simulink library "MainLibrary"  (R2022b)
settings: Solver=VariableStepAuto  StartTime=0.0  StopTime=10.0  RelTol=1e-3
undefined symbols (not defined in the file or in its folder): Data, Data_SL_Info, Encoding, Encoding_SL_Info, Height, IsBigendian, Step, Width
libraries: robotlib x14, simulink_extras x2, robotcorelib x1
settings Model: Creator=20211327  LastModifiedBy=20222146

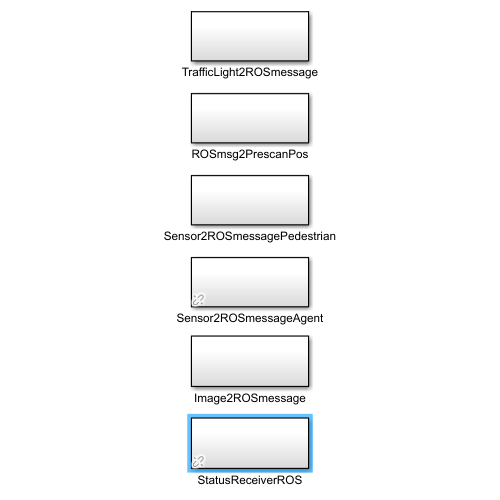
[thumbnail: Simulink's stored preview of the top-level diagram]
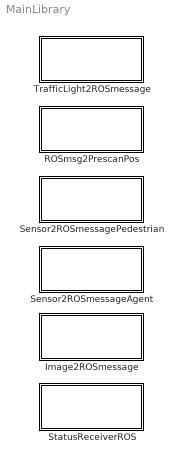
== system MainLibrary ==
  Image2ROSmessage : Subsystem
  ROSmsg2PrescanPos : Subsystem
  Sensor2ROSmessageAgent : Subsystem  AncestorBlock=MainLibrary/Sensor2ROSmessage
      settings: LibrarySourceBlock=MainLibrary/Sensor2ROSmessage
  Sensor2ROSmessagePedestrian : Subsystem
  StatusReceiverROS : Subsystem  AncestorBlock=MainLibrary/Image2ROSmessage
      settings: LibrarySourceBlock=MainLibrary/Image2ROSmessage
  TrafficLight2ROSmessage : Subsystem

== system MainLibrary/Image2ROSmessage ==
  Image Publisher : Subsystem  mask(Image publisher block){}
      mask help: This block publishes the camera image output of the experiment to a ros topic
      mask Display:
      | fprintf('Image Publisher')
      | port_label('input',1,'R')
      | port_label('input',2,'G')
      | port_label('input',3,'B')

== system MainLibrary/ROSmsg2PrescanPos ==
  ROS msg to Prescan Pos : Subsystem

== system MainLibrary/Sensor2ROSmessageAgent ==
  Sensor ROS Message Agent : Subsystem  AncestorBlock=MainLibrary/Sensor2ROSmessagePedestrian/Sensor ROS Message Pedestrian  TreatAsAtomicUnit=on
      settings: LibrarySourceBlock=MainLibrary/Sensor2ROSmessagePedestrian/Sensor ROS Message Pedestrian

== system MainLibrary/Sensor2ROSmessagePedestrian ==
  Sensor ROS Message Pedestrian : Subsystem  TreatAsAtomicUnit=on

== system MainLibrary/StatusReceiverROS ==
  Status Receiver ROS : Subsystem

== system MainLibrary/TrafficLight2ROSmessage ==
  Traffic Light ROS Message : Subsystem

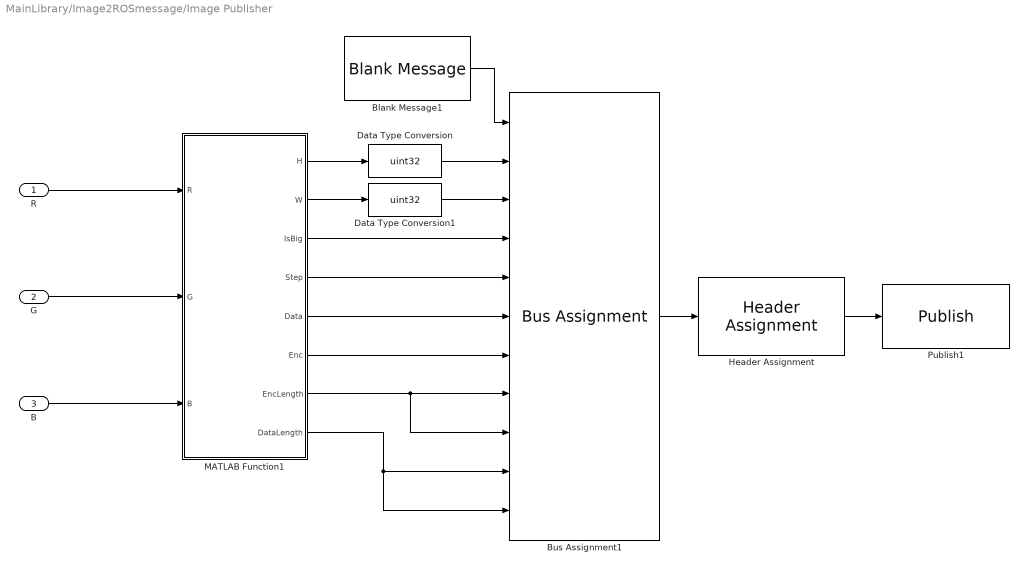
== system MainLibrary/Image2ROSmessage/Image Publisher ==
  R : Inport
  G : Inport  Port=2
  B : Inport  Port=3
  Blank Message1 : robotlib/Blank Message  messageClass=Message  entityType=sensor_msgs/Image  messageType=sensor_msgs/Image  SampleTime=inf  legacyBusStruct=off
  Bus Assignment1 : BusAssignment  AssignedSignals=Height,Width,IsBigendian,Step,Data,Encoding,Encoding_SL_Info.CurrentLength,Encoding_SL_Info.ReceivedLength,Data_SL_Info.CurrentLength,Data_SL_Info.ReceivedLength
  Data Type Conversion : DataTypeConversion  OutDataTypeStr=uint32  RndMeth=Round  SaturateOnIntegerOverflow=off
  Data Type Conversion1 : DataTypeConversion  OutDataTypeStr=uint32  RndMeth=Round  SaturateOnIntegerOverflow=off
  Header Assignment : robotlib/Header Assignment  SetFrameID=on  FrameID=camera  InsertTimeStamp=on  SetHeaderFieldName=Use the default Header field name  HeaderFieldName=Header
  MATLAB Function1 : MATLAB Function  TreatAsAtomicUnit=on
  Publish1 : robotlib/Publish  topicSource=Specify your own  topic=/camera/image  messageType=sensor_msgs/Image  legacyBusStruct=off  messageQueueLength=1
  wires:
  R/1 -> MATLAB Function1/1(R)
  G/1 -> MATLAB Function1/2(G)
  B/1 -> MATLAB Function1/3(B)
  Data Type Conversion/1 -> Bus Assignment1/2
  Data Type Conversion1/1 -> Bus Assignment1/3
  Bus Assignment1/1 -> Header Assignment/1
  Header Assignment/1 -> Publish1/1
  MATLAB Function1/4(Step) -> Bus Assignment1/5
  MATLAB Function1/7(EncLength) -> Bus Assignment1/9, Bus Assignment1/8
  MATLAB Function1/3(IsBig) -> Bus Assignment1/4
  MATLAB Function1/2(W) -> Data Type Conversion1/1
  MATLAB Function1/5(Data) -> Bus Assignment1/6
  Blank Message1/1 -> Bus Assignment1/1
  MATLAB Function1/6(Enc) -> Bus Assignment1/7
  MATLAB Function1/1(H) -> Data Type Conversion/1
  MATLAB Function1/8(DataLength) -> Bus Assignment1/11, Bus Assignment1/10

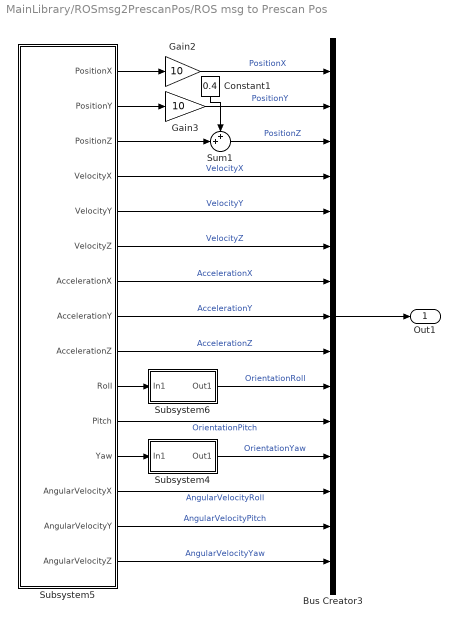
== system MainLibrary/ROSmsg2PrescanPos/ROS msg to Prescan Pos ==
  Bus Creator3 : BusCreator  Inputs=15  OutDataTypeStr=Bus: PRESCAN_STATEACTUATORDATA  NonVirtualBus=on
  Constant1 : Constant  Value=0.4
  Gain2 : Gain  Gain=10
  Gain3 : Gain  Gain=10
  Subsystem4 : Subsystem
  Subsystem5 : Subsystem
  Subsystem6 : Subsystem
  Sum1 : Sum  Inputs=++|
  Out1 : Outport
  wires:
  Subsystem5/15(AngularVelocityZ) -> Bus Creator3/15  "AngularVelocityYaw"
  Subsystem5/3(PositionZ) -> Sum1/2
  Subsystem5/7("AccelerationX ") -> Bus Creator3/7  "AccelerationX"
  Gain3/1 -> Bus Creator3/2  "PositionY"
  Subsystem5/14(AngularVelocityY) -> Bus Creator3/14  "AngularVelocityPitch"
  Subsystem5/8(AccelerationY) -> Bus Creator3/8  "AccelerationY"
  Subsystem5/5(VelocityY) -> Bus Creator3/5  "VelocityY"
  Subsystem5/6(VelocityZ) -> Bus Creator3/6  "VelocityZ"
  Subsystem5/2(PositionY) -> Gain3/1
  Subsystem5/10(Roll) -> Subsystem6/1(In1)
  Subsystem4/1(Out1) -> Bus Creator3/12  "OrientationYaw"
  Gain2/1 -> Bus Creator3/1  "PositionX"
  Subsystem5/4(VelocityX) -> Bus Creator3/4  "VelocityX"
  Sum1/1 -> Bus Creator3/3  "PositionZ"
  Subsystem5/13(AngularVelocityX) -> Bus Creator3/13  "AngularVelocityRoll"
  Constant1/1 -> Sum1/1
  Subsystem5/11(Pitch) -> Bus Creator3/11  "OrientationPitch"
  Subsystem5/1(PositionX) -> Gain2/1
  Subsystem6/1(Out1) -> Bus Creator3/10  "OrientationRoll"
  Subsystem5/12(Yaw) -> Subsystem4/1(In1)
  Bus Creator3/1 -> Out1/1
  Subsystem5/9(AccelerationZ) -> Bus Creator3/9  "AccelerationZ"

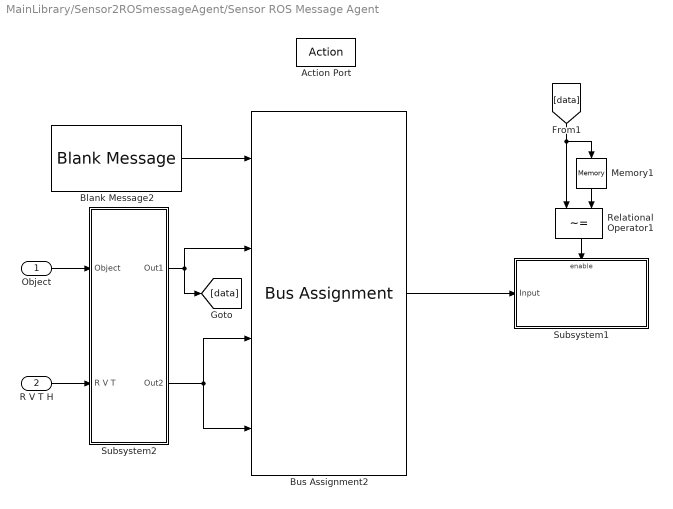
== system MainLibrary/Sensor2ROSmessageAgent/Sensor ROS Message Agent ==
  Object : Inport
  R V T H : Inport  Port=2
  Action Port : ActionPort
  Blank Message2 : robotlib/Blank Message  messageClass=Message  entityType=std_msgs/String  messageType=std_msgs/String  SampleTime=inf  legacyBusStruct=off
  Bus Assignment2 : BusAssignment  AssignedSignals=Data,Data_SL_Info.CurrentLength,Data_SL_Info.ReceivedLength
  Memory1 : Memory  InitialCondition=zeros(1,128)  InheritSampleTime=on
  Relational Operator1 : RelationalOperator  Operator=~=  OutDataTypeStr=boolean  RndMeth=Simplest  InputSameDT=off
  Subsystem1 : Subsystem
  Subsystem2 : Subsystem  AncestorBlock=MainLibrary/Sensor2ROSmessagePedestrian/Sensor ROS Message Pedestrian/Subsystem2
      settings: LibrarySourceBlock=MainLibrary/Sensor2ROSmessagePedestrian/Sensor ROS Message Pedestrian/Subsystem2
  wires:
  Bus Assignment2/1 -> Subsystem1/1(Input)
  Blank Message2/1 -> Bus Assignment2/1
  Memory1/1 -> Relational Operator1/2
  [data] -> Memory1/1, Relational Operator1/1
  Relational Operator1/1 -> Subsystem1/Enable
  Subsystem2/2(Out2) -> Bus Assignment2/4, Bus Assignment2/3
  Object/1 -> Subsystem2/1(Object)
  R V T H/1 -> Subsystem2/2(R V T)
  Subsystem2/1(Out1) -> Bus Assignment2/2, [data]

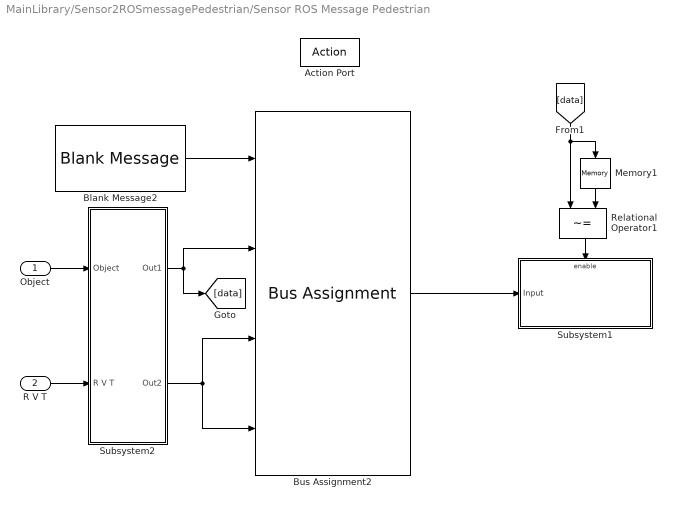
== system MainLibrary/Sensor2ROSmessagePedestrian/Sensor ROS Message Pedestrian ==
  Object : Inport
  R V T : Inport  Port=2
  Action Port : ActionPort
  Blank Message2 : robotlib/Blank Message  messageClass=Message  entityType=std_msgs/String  messageType=std_msgs/String  SampleTime=inf  legacyBusStruct=off
  Bus Assignment2 : BusAssignment  AssignedSignals=Data,Data_SL_Info.CurrentLength,Data_SL_Info.ReceivedLength
  Memory1 : Memory  InitialCondition=zeros(1,128)  InheritSampleTime=on
  Relational Operator1 : RelationalOperator  Operator=~=  OutDataTypeStr=boolean  RndMeth=Simplest  InputSameDT=off
  Subsystem1 : Subsystem
  Subsystem2 : Subsystem
  wires:
  Subsystem2/2(Out2) -> Bus Assignment2/3, Bus Assignment2/4
  Bus Assignment2/1 -> Subsystem1/1(Input)
  Subsystem2/1(Out1) -> Bus Assignment2/2, [data]
  Blank Message2/1 -> Bus Assignment2/1
  R V T/1 -> Subsystem2/2(R V T)
  Object/1 -> Subsystem2/1(Object)
  Memory1/1 -> Relational Operator1/2
  [data] -> Memory1/1, Relational Operator1/1
  Relational Operator1/1 -> Subsystem1/Enable

== system MainLibrary/StatusReceiverROS/Status Receiver ROS ==
  Blank Message : robotlib/Blank Message  messageClass=Message  entityType=std_msgs/Bool  messageType=std_msgs/Bool  SampleTime=inf  legacyBusStruct=off
  Bus tf3 : BusAssignment  AssignedSignals=Data
  Constant : Constant  OutDataTypeStr=boolean
  Publish : robotlib/Publish  topicSource=Specify your own  topic=/status  messageType=std_msgs/Bool  legacyBusStruct=off  messageQueueLength=1
  wires:
  Bus tf3/1 -> Publish/1
  Constant/1 -> Bus tf3/2
  Blank Message/1 -> Bus tf3/1

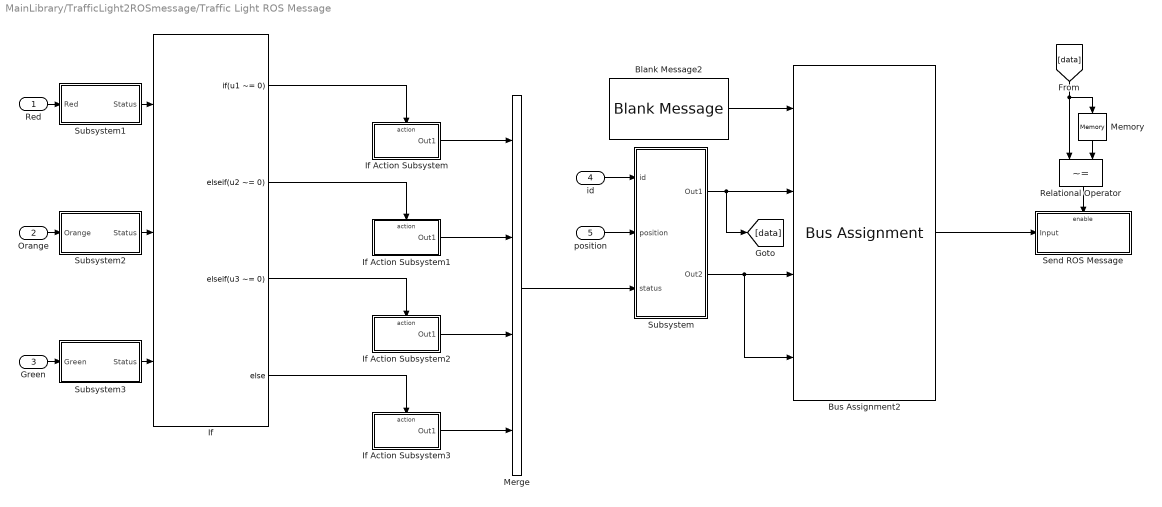
== system MainLibrary/TrafficLight2ROSmessage/Traffic Light ROS Message ==
  Red : Inport
  Orange : Inport  Port=2
  Green : Inport  Port=3
  id : Inport  Port=4
  position : Inport  Port=5
  Blank Message2 : robotlib/Blank Message  messageClass=Message  entityType=std_msgs/String  messageType=std_msgs/String  SampleTime=inf  legacyBusStruct=off
  Bus Assignment2 : BusAssignment  AssignedSignals=Data,Data_SL_Info.CurrentLength,Data_SL_Info.ReceivedLength
  If : If  NumInputs=3  IfExpression=u1 ~= 0  ElseIfExpressions=u2 ~= 0, u3 ~= 0
  If Action Subsystem : Subsystem  TreatAsAtomicUnit=on
  If Action Subsystem1 : Subsystem  TreatAsAtomicUnit=on
  If Action Subsystem2 : Subsystem  TreatAsAtomicUnit=on
  If Action Subsystem3 : Subsystem  TreatAsAtomicUnit=on
  Memory : Memory  InitialCondition=zeros(1,128)
  Merge : Merge  Inputs=4
  Relational Operator : RelationalOperator  Operator=~=  OutDataTypeStr=boolean  RndMeth=Simplest  InputSameDT=off
  Send ROS Message : Subsystem  TreatAsAtomicUnit=on
  Subsystem : Subsystem
  Subsystem1 : Subsystem
  Subsystem2 : Subsystem
  Subsystem3 : Subsystem
  wires:
  Subsystem/1(Out1) -> [data], Bus Assignment2/2
  Subsystem/2(Out2) -> Bus Assignment2/4, Bus Assignment2/3
  Blank Message2/1 -> Bus Assignment2/1
  Merge/1 -> Subsystem/3(status)
  Relational Operator/1 -> Send ROS Message/Enable
  Memory/1 -> Relational Operator/2
  Bus Assignment2/1 -> Send ROS Message/1(Input)
  id/1 -> Subsystem/1(id)
  position/1 -> Subsystem/2(position)
  [data] -> Relational Operator/1, Memory/1
  If/3 -> If Action Subsystem2/Action
  If Action Subsystem2/1(Out1) -> Merge/3
  If Action Subsystem/1(Out1) -> Merge/1
  If/4 -> If Action Subsystem3/Action
  If Action Subsystem3/1(Out1) -> Merge/4
  If/2 -> If Action Subsystem1/Action
  If/1 -> If Action Subsystem/Action
  If Action Subsystem1/1(Out1) -> Merge/2
  Subsystem1/1(Status) -> If/1
  Red/1 -> Subsystem1/1(Red)
  Subsystem2/1(Status) -> If/2
  Subsystem3/1(Status) -> If/3
  Green/1 -> Subsystem3/1(Green)
  Orange/1 -> Subsystem2/1(Orange)

== system MainLibrary/ROSmsg2PrescanPos/ROS msg to Prescan Pos/Subsystem4 ==
  In1 : Inport
  Constant : Constant  Value=0
  Degrees to Radians : simulink_extras/Transformations/Degrees to Radians
  Sum : Sum  Inputs=|++
  Out1 : Outport
  wires:
  Degrees to Radians/1 -> Sum/1
  Sum/1 -> Out1/1
  In1/1 -> Sum/2
  Constant/1 -> Degrees to Radians/1

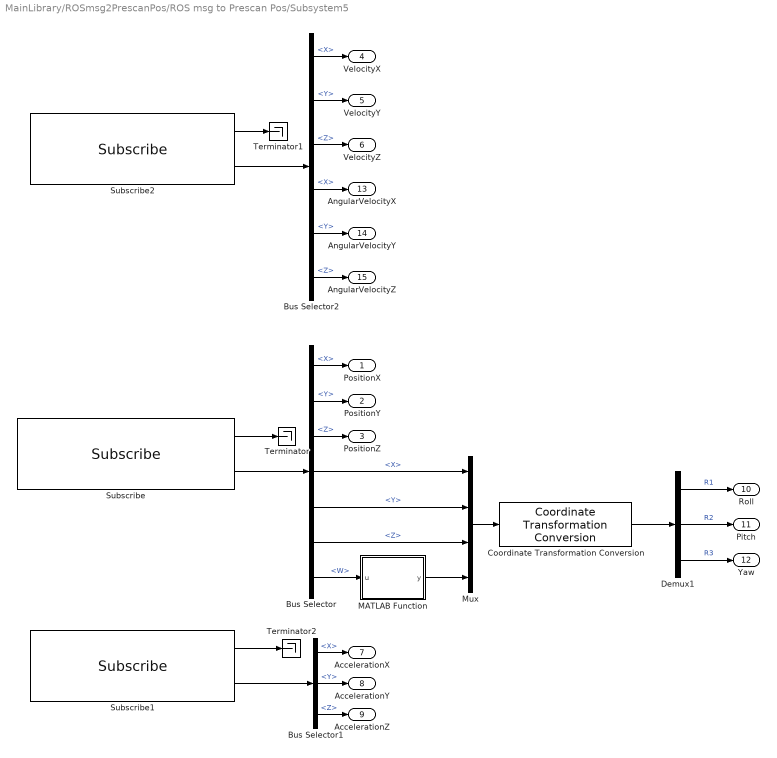
== system MainLibrary/ROSmsg2PrescanPos/ROS msg to Prescan Pos/Subsystem5 ==
  Bus Selector : BusSelector  OutputSignals=Pose.Position.X,Pose.Position.Y,Pose.Position.Z,Pose.Orientation.X,Pose.Orientation.Y,Pose.Orientation.Z,Pose.Orientation.W
  Bus Selector1 : BusSelector  OutputSignals=Twist.Linear.X,Twist.Linear.Y,Twist.Linear.Z
  Bus Selector2 : BusSelector  OutputSignals=Twist.Linear.X,Twist.Linear.Y,Twist.Linear.Z,Twist.Angular.X,Twist.Angular.Y,Twist.Angular.Z
  Coordinate Transformation Conversion : robotcorelib/Coordinate Transformation Conversion  InputRepresentation=Quaternion  InputEulerSequence=XYZ  ShowTrVecInputPort=on  OutputRepresentation=Euler Angles  OutputEulerSequence=ZYX  ShowTrVecOutputPort=on  SimulateUsing=Interpreted execution
  Demux1 : Demux  Outputs=3
  MATLAB Function : MATLAB Function  TreatAsAtomicUnit=on
  Mux : Mux
  Subscribe : robotlib/Subscribe  topicSource=Specify your own  topic=/vrpn_client_node/Car_2_Tracking/pose  messageType=geometry_msgs/PoseStamped  SampleTime=-1  legacyBusStruct=off  messageQueueLength=1
  Subscribe1 : robotlib/Subscribe  topicSource=Select from ROS network  topic=/vrpn_client_node/Car_3_Tracking/accel  messageType=geometry_msgs/TwistStamped  SampleTime=-1  legacyBusStruct=off  messageQueueLength=1
  Subscribe2 : robotlib/Subscribe  topicSource=Select from ROS network  topic=/vrpn_client_node/Car_3_Tracking/twist  messageType=geometry_msgs/TwistStamped  SampleTime=-1  legacyBusStruct=off  messageQueueLength=1
  Terminator : Terminator
  Terminator1 : Terminator
  Terminator2 : Terminator
  PositionX : Outport
  PositionY : Outport  Port=2
  PositionZ : Outport  Port=3
  VelocityX : Outport  Port=4
  VelocityY : Outport  Port=5
  VelocityZ : Outport  Port=6
  "AccelerationX " : Outport  Port=7
  AccelerationY : Outport  Port=8
  AccelerationZ : Outport  Port=9
  Roll : Outport  Port=10
  Pitch : Outport  Port=11
  Yaw : Outport  Port=12
  AngularVelocityX : Outport  Port=13
  AngularVelocityY : Outport  Port=14
  AngularVelocityZ : Outport  Port=15
  wires:
  Bus Selector2/3 -> VelocityZ/1  "<Z>"
  Subscribe2/1 -> Terminator1/1
  Bus Selector/7 -> MATLAB Function/1(u)  "<W>"
  Bus Selector/4 -> Mux/1  "<X>"
  Subscribe/1 -> Terminator/1
  Subscribe2/2 -> Bus Selector2/1
  Bus Selector2/6 -> AngularVelocityZ/1  "<Z>"
  Bus Selector1/3 -> AccelerationZ/1  "<Z>"
  Subscribe1/2 -> Bus Selector1/1
  Bus Selector2/2 -> VelocityY/1  "<Y>"
  Bus Selector2/4 -> AngularVelocityX/1  "<X>"
  Bus Selector/5 -> Mux/2  "<Y>"
  Bus Selector1/2 -> AccelerationY/1  "<Y>"
  Demux1/2 -> Pitch/1  "R2"
  Subscribe1/1 -> Terminator2/1
  Bus Selector/6 -> Mux/3  "<Z>"
  Demux1/3 -> Yaw/1  "R3"
  Subscribe/2 -> Bus Selector/1
  Mux/1 -> Coordinate Transformation Conversion/1
  Bus Selector2/5 -> AngularVelocityY/1  "<Y>"
  Bus Selector/3 -> PositionZ/1  "<Z>"
  Bus Selector2/1 -> VelocityX/1  "<X>"
  Bus Selector/2 -> PositionY/1  "<Y>"
  Bus Selector1/1 -> "AccelerationX "/1  "<X>"
  Demux1/1 -> Roll/1  "R1"
  Bus Selector/1 -> PositionX/1  "<X>"
  MATLAB Function/1(y) -> Mux/4
  Coordinate Transformation Conversion/1 -> Demux1/1

== system MainLibrary/ROSmsg2PrescanPos/ROS msg to Prescan Pos/Subsystem6 ==
  In1 : Inport
  Constant : Constant  Value=180
  Degrees to Radians : simulink_extras/Transformations/Degrees to Radians
  Sum : Sum  Inputs=|++
  Out1 : Outport
  wires:
  Degrees to Radians/1 -> Sum/1
  Sum/1 -> Out1/1
  In1/1 -> Sum/2
  Constant/1 -> Degrees to Radians/1

== system MainLibrary/Sensor2ROSmessageAgent/Sensor ROS Message Agent/Subsystem1 ==
  Input : Inport
  Enable : EnablePort
  Publish2 : robotlib/Publish  topicSource=Specify your own  topic=/Pedestrian  messageType=std_msgs/String  legacyBusStruct=off  messageQueueLength=1
  wires:
  Input/1 -> Publish2/1

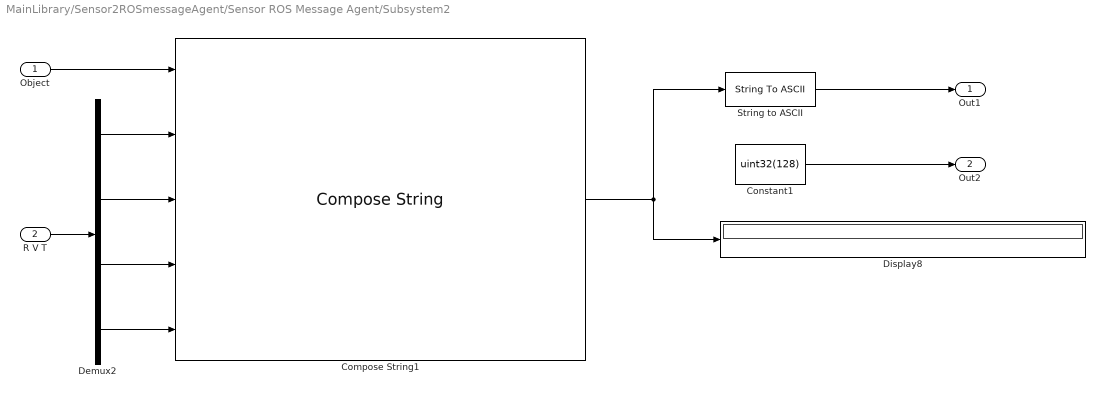
== system MainLibrary/Sensor2ROSmessageAgent/Sensor ROS Message Agent/Subsystem2 ==
  Object : Inport
  R V T : Inport  Port=2
  Compose String1 : ComposeString  Format="\"{'id': '%s', 'range': %.4f, 'vel': %.4f, 'theta': %.4f,'heading': %.4f}\""
  Constant1 : Constant  Value=uint32(128)
  Demux2 : Demux
  Display8 : Display
  String to ASCII : StringToASCII  OutputVectorSize=128
  Out1 : Outport
  Out2 : Outport  Port=2
  wires:
  Compose String1/1 -> Display8/1, String to ASCII/1
  R V T/1 -> Demux2/1
  Constant1/1 -> Out2/1
  String to ASCII/1 -> Out1/1
  Object/1 -> Compose String1/1
  Demux2/1 -> Compose String1/2
  Demux2/2 -> Compose String1/3
  Demux2/3 -> Compose String1/4
  Demux2/4 -> Compose String1/5

== system MainLibrary/Sensor2ROSmessagePedestrian/Sensor ROS Message Pedestrian/Subsystem1 ==
  Input : Inport
  Enable : EnablePort
  Publish2 : robotlib/Publish  topicSource=Specify your own  topic=/Pedestrian  messageType=std_msgs/String  legacyBusStruct=off  messageQueueLength=1
  wires:
  Input/1 -> Publish2/1

== system MainLibrary/Sensor2ROSmessagePedestrian/Sensor ROS Message Pedestrian/Subsystem2 ==
  Object : Inport
  R V T : Inport  Port=2
  Compose String1 : ComposeString  Format="\"{'id': 'pd_%.0f', 'range': %.4f, 'vel': %.4f, 'theta': %.4f}\""
  Constant1 : Constant  Value=uint32(128)
  Demux2 : Demux  Outputs=3
  Display8 : Display
  String to ASCII : StringToASCII  OutputVectorSize=128
  Out1 : Outport
  Out2 : Outport  Port=2
  wires:
  Compose String1/1 -> Display8/1, String to ASCII/1
  R V T/1 -> Demux2/1
  Constant1/1 -> Out2/1
  String to ASCII/1 -> Out1/1
  Object/1 -> Compose String1/1
  Demux2/1 -> Compose String1/2
  Demux2/2 -> Compose String1/3
  Demux2/3 -> Compose String1/4

== system MainLibrary/TrafficLight2ROSmessage/Traffic Light ROS Message/If Action Subsystem ==
  Action Port : ActionPort  ActionPortLabel=if(u1 ~= 0)
  String Constant : StringConstant  String="\"red\""
  Out1 : Outport
  wires:
  String Constant/1 -> Out1/1

== system MainLibrary/TrafficLight2ROSmessage/Traffic Light ROS Message/If Action Subsystem1 ==
  Action Port : ActionPort  ActionPortLabel=elseif(u2 ~= 0)
  String Constant : StringConstant  String="\"orange\""
  Out1 : Outport
  wires:
  String Constant/1 -> Out1/1

== system MainLibrary/TrafficLight2ROSmessage/Traffic Light ROS Message/If Action Subsystem2 ==
  Action Port : ActionPort  ActionPortLabel=elseif( u3 ~= 0)
  String Constant : StringConstant  String="\"green\""
  Out1 : Outport
  wires:
  String Constant/1 -> Out1/1

== system MainLibrary/TrafficLight2ROSmessage/Traffic Light ROS Message/If Action Subsystem3 ==
  Action Port : ActionPort  ActionPortLabel=else
  String Constant : StringConstant  String="\"colourless\""
  Out1 : Outport
  wires:
  String Constant/1 -> Out1/1

== system MainLibrary/TrafficLight2ROSmessage/Traffic Light ROS Message/Send ROS Message ==
  Input : Inport
  Enable : EnablePort
  Publish2 : robotlib/Publish  topicSource=Specify your own  topic=/traffic_light  messageType=std_msgs/String  legacyBusStruct=off  messageQueueLength=1
  wires:
  Input/1 -> Publish2/1

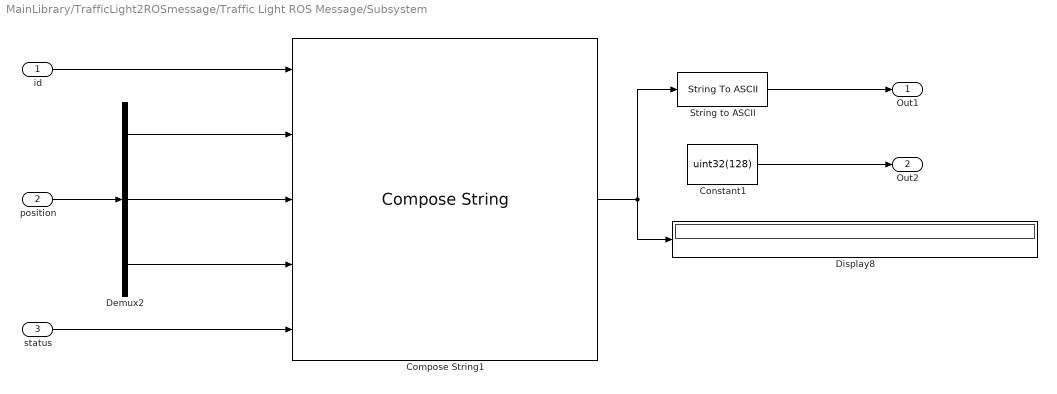
== system MainLibrary/TrafficLight2ROSmessage/Traffic Light ROS Message/Subsystem ==
  id : Inport
  position : Inport  Port=2
  status : Inport  Port=3
  Compose String1 : ComposeString  Format="\"{'id': 'tl_%s', 'position': [%.4f, %.4f, %.4f], 'status': '%s'}\""
  Constant1 : Constant  Value=uint32(128)
  Demux2 : Demux  Outputs=3
  Display8 : Display
  String to ASCII : StringToASCII  OutputVectorSize=128
  Out1 : Outport
  Out2 : Outport  Port=2
  wires:
  position/1 -> Demux2/1
  Compose String1/1 -> Display8/1, String to ASCII/1
  Demux2/2 -> Compose String1/3
  Demux2/1 -> Compose String1/2
  Demux2/3 -> Compose String1/4
  String to ASCII/1 -> Out1/1
  Constant1/1 -> Out2/1
  status/1 -> Compose String1/5
  id/1 -> Compose String1/1

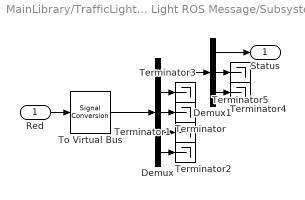
== system MainLibrary/TrafficLight2ROSmessage/Traffic Light ROS Message/Subsystem1 ==
  Red : Inport
  Demux : Demux  Outputs=5
  Demux1 : Demux  Outputs=3
  Terminator{,1..5} (6 alike) : Terminator
  To Virtual Bus : SignalConversion  ConversionOutput=Virtual bus  OverrideOpt=off
  Status : Outport
  wires:
  Demux1/3 -> Terminator4/1
  Demux/3 -> Terminator/1
  Demux/2 -> Terminator3/1
  To Virtual Bus/1 -> Demux/1
  Demux/4 -> Terminator1/1
  Demux/1 -> Demux1/1
  Demux/5 -> Terminator2/1
  Demux1/2 -> Terminator5/1
  Demux1/1 -> Status/1
  Red/1 -> To Virtual Bus/1

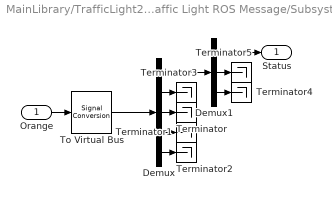
== system MainLibrary/TrafficLight2ROSmessage/Traffic Light ROS Message/Subsystem2 ==
  Orange : Inport
  Demux : Demux  Outputs=5
  Demux1 : Demux  Outputs=3
  Terminator{,1..5} (6 alike) : Terminator
  To Virtual Bus : SignalConversion  ConversionOutput=Virtual bus  OverrideOpt=off
  Status : Outport
  wires:
  Demux/4 -> Terminator1/1
  Demux/3 -> Terminator/1
  Demux1/2 -> Terminator5/1
  To Virtual Bus/1 -> Demux/1
  Demux/1 -> Demux1/1
  Demux/2 -> Terminator3/1
  Demux/5 -> Terminator2/1
  Demux1/3 -> Terminator4/1
  Demux1/1 -> Status/1
  Orange/1 -> To Virtual Bus/1

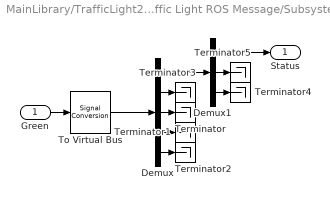
== system MainLibrary/TrafficLight2ROSmessage/Traffic Light ROS Message/Subsystem3 ==
  Green : Inport
  Demux : Demux  Outputs=5
  Demux1 : Demux  Outputs=3
  Terminator{,1..5} (6 alike) : Terminator
  To Virtual Bus : SignalConversion  ConversionOutput=Virtual bus  OverrideOpt=off
  Status : Outport
  wires:
  Demux1/1 -> Status/1
  Demux1/2 -> Terminator5/1
  To Virtual Bus/1 -> Demux/1
  Demux/3 -> Terminator/1
  Green/1 -> To Virtual Bus/1
  Demux/1 -> Demux1/1
  Demux1/3 -> Terminator4/1
  Demux/5 -> Terminator2/1
  Demux/4 -> Terminator1/1
  Demux/2 -> Terminator3/1

== matlab function MainLibrary/Image2ROSmessage/Image Publisher/MATLAB Function1 ==
  data: R input; G input; B input; H output; W output; IsBig output; Step output; Data output; Enc output; EncLength output; DataLength output
% function [RGB_matrix,encoding,height,width] = RGB2ROS(R,G,B)
% function [imgMatrix] = RGB2ROS(R,G,B)
function [H, W, IsBig, Step, Data, Enc, EncLength, DataLength] = fcn(R,G,B)

RGBmatrix = cat(3,R,G,B);
[H, W, n] = size(RGBmatrix);

im = permute(RGBmatrix,[2 1 3]);
Data1 = im(:);
Data2 = reshape(Data1,[H*W,n])';
Data = Data2(:);

Enc = zeros(1,128, 'uint8');
Enc(1:4) = uint8('rgb8'); %   uint8('rgb8')
EncLength = uint32(4);

IsBig = uint8(0);
Step = uint32(W*n);

DataLength = uint32(H*W*n);

end

== matlab function MainLibrary/ROSmsg2PrescanPos/ROS msg to Prescan Pos/Subsystem5/MATLAB Function ==
  data: u input; y output
function y = fcn(u)
    if u == 0
        y = 1;
    else
        y = u;
    end
